simulink model "Motor_Pos"  (Simulink 7.9)
settings: Solver=ode15s  StartTime=0.0  StopTime=0.2  RelTol=1e-3
undefined symbols (not defined in the file): b, J, K, L, R
settings Model: Creator=maen  LastModifiedBy=Rick
settings DebuggingCC: FcnCallInpInsideContextMsg=Use local settings
settings GRTTargetCC: CombineOutputUpdateFcns=off  GRTInterface=on

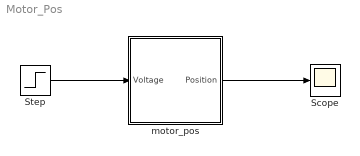
== system Motor_Pos ==
  Scope : Scope
      settings: TimeRange=0.2  YMin=0  YMax=10
  Step : Step  Time=0  SampleTime=0
  motor_pos : Subsystem
  wires:
  Step/1 -> motor_pos/1(Voltage)
  motor_pos/1(Position) -> Scope/1

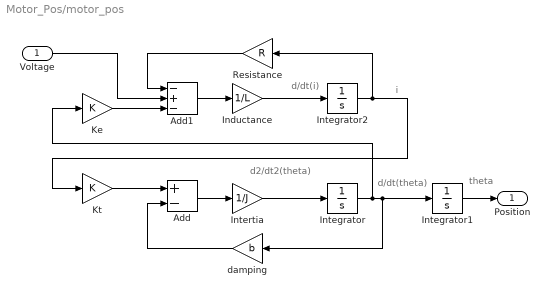
== system Motor_Pos/motor_pos ==
  note: i
  note: d/dt(theta)
  note: d2/dt2(theta)
  note: d/dt(i)
  note: theta
  Voltage : Inport
  Add : Sum  Inputs=+-
  Add1 : Sum  Inputs=-+-
  Inductance : Gain  Gain=1/L
  Integrator : Integrator
  Integrator1 : Integrator
  Integrator2 : Integrator
  Intertia : Gain  Gain=1/J
  Ke : Gain  Gain=K
  Kt : Gain  Gain=K
  Resistance : Gain  Gain=R
  damping : Gain  Gain=b
  Position : Outport
  wires:
  Inductance/1 -> Integrator2/1
  Integrator/1 -> Integrator1/1, damping/1, Ke/1
  Integrator1/1 -> Position/1
  Intertia/1 -> Integrator/1
  Integrator2/1 -> Kt/1, Resistance/1
  Add/1 -> Intertia/1
  Add1/1 -> Inductance/1
  Kt/1 -> Add/1
  damping/1 -> Add/2
  Ke/1 -> Add1/3
  Resistance/1 -> Add1/1
  Voltage/1 -> Add1/2
